simulink model "Rebuild"  (R2024b)
settings: Solver=VariableStepAuto  StartTime=0.0  StopTime=12  RelTol=1e-3
values from neighbouring files (symbols this model uses):
  A = 1.1    [RT14e_Parameters.m]    (also in RT15e_Parameters.m = 1.088; RT15evo_Parameters.m = 1.088)
  Aero_balance = 55    [RT14e_Parameters.m]    (also in RT15e_Parameters.m; RT15evo_Parameters.m)
  Aeromaps_ON = 0    [SIM_setup.m]
  air_density = 1.2    [SIM_setup.m]
  Balance_FW = Data_FW_STD(1:end,2)    [RT15e_Parameters.m]    (also in RT15evo_Parameters.m)
  Balance_R_11 = Data_R_11(1:end,2)    [RT15e_Parameters.m]    (also in RT15evo_Parameters.m)
  Br_coef_of_friction_F = 0.33    [RT14e_Parameters.m]    (also in RT15e_Parameters.m; RT15evo_Parameters.m)
  Br_coef_of_friction_R = 0.33    [RT14e_Parameters.m]    (also in RT15e_Parameters.m; RT15evo_Parameters.m)
  Br_pistons_area_F = 3617.26/1e6    (= 0.00361726)    [RT14e_Parameters.m]    (also in RT15e_Parameters.m; RT15evo_Parameters.m)
  Br_pistons_area_R = 2026.83/1e6    (= 0.00202683)    [RT14e_Parameters.m]    (also in RT15e_Parameters.m; RT15evo_Parameters.m)
  CdA = 1.31*A    (= 1.441)    [RT14e_Parameters.m]    (also in RT15e_Parameters.m = 1.700544; RT15evo_Parameters.m = 1.700544)
  CdA_FW = Data_FW_STD(1:end,3)    [RT15e_Parameters.m]    (also in RT15evo_Parameters.m)
  CdA_R_11 = Data_R_11(1:end,3)    [RT15e_Parameters.m]    (also in RT15evo_Parameters.m)
  ClA = 3.3*A    (= 3.63)    [RT14e_Parameters.m]    (also in RT15e_Parameters.m = 4.36288; RT15evo_Parameters.m = 4.36288)
  ClA_FW = Data_FW_STD(1:end,4)    [RT15e_Parameters.m]    (also in RT15evo_Parameters.m)
  ClA_R_11 = Data_R_11(1:end,4)    [RT15e_Parameters.m]    (also in RT15evo_Parameters.m)
  CoG_z = 0.35    [RT14e_Parameters.m]    (also in RT15e_Parameters.m = 0.28495; RT15evo_Parameters.m = 0.28495)
  Default_Fz_FL = Default_Fz_F/2 + (Default_Fz_F*CoG_y/Track_Front)    [RT14e_Parameters.m]    (also in RT15e_Parameters.m; RT15evo_Parameters.m)
  Default_Fz_FR = Default_Fz_F/2 - (Default_Fz_F*CoG_y/Track_Front)    [RT14e_Parameters.m]    (also in RT15e_Parameters.m; RT15evo_Parameters.m)
  Default_Fz_RL = Default_Fz_R/2 + (Default_Fz_R*CoG_y/Track_Rear)    [RT14e_Parameters.m]    (also in RT15e_Parameters.m; RT15evo_Parameters.m)
  Default_Fz_RR = Default_Fz_R/2 - (Default_Fz_R*CoG_y/Track_Rear)    [RT14e_Parameters.m]    (also in RT15e_Parameters.m; RT15evo_Parameters.m)
  Effective_br_disk_r_F = 0.0905    [RT14e_Parameters.m]    (also in RT15e_Parameters.m; RT15evo_Parameters.m)
  Effective_br_disk_r_R = 0.0895    [RT14e_Parameters.m]    (also in RT15e_Parameters.m; RT15evo_Parameters.m)
  Front_brake_balance = 0.0    (= 0)    [RT14e_Parameters.m]    (also in RT15e_Parameters.m; RT15evo_Parameters.m)
  Front_brake_pump_area = 153.94    [RT14e_Parameters.m]    (also in RT15e_Parameters.m; RT15evo_Parameters.m)
  Front_desired_brake_p_balance = 0.6    [RT14e_Parameters.m]    (also in RT15e_Parameters.m; RT15evo_Parameters.m)
  FW_Setup = Data_FW_STD(1:end,1)    [RT15e_Parameters.m]    (also in RT15evo_Parameters.m)
  Fx = Data_Fx(2:end,3:end)    [RT14e_Parameters.m]    (also in RT15e_Parameters.m; RT15evo_Parameters.m)
  Fy = Data_Fy(2:end,3:end)    [RT14e_Parameters.m]    (also in RT15e_Parameters.m; RT15evo_Parameters.m)
  Fz = Data_Fy(2:end,2)    [RT14e_Parameters.m]    (also in RT15e_Parameters.m; RT15evo_Parameters.m)
  g = 9.81    [SIM_setup.m]
  Gear_ratio = 12.9    [RT14e_Parameters.m]    (also in RT15e_Parameters.m; RT15evo_Parameters.m)
  Iz_wehicle = 120    [RT14e_Parameters.m]    (also in RT15e_Parameters.m; RT15evo_Parameters.m)
  Iz_wheel = 0.15    [RT14e_Parameters.m]    (also in RT15e_Parameters.m; RT15evo_Parameters.m)
  Lf = Wheelbase - CoG_x    (= 0.77)    [RT14e_Parameters.m]    (also in RT15e_Parameters.m = 0.7504; RT15evo_Parameters.m = 0.7504)
  LLTD = 0.45    [RT14e_Parameters.m]    (also in RT15e_Parameters.m = 0.55; RT15evo_Parameters.m = 0.55)
  Lock_brake_balance = false    [RT14e_Parameters.m]    (also in RT15e_Parameters.m; RT15evo_Parameters.m)
  Lr = Wheelbase - Lf    (= 0.755)    [RT14e_Parameters.m]    (also in RT15e_Parameters.m = 0.7746; RT15evo_Parameters.m = 0.7746)
  Mass = Vehicle_mass + Driver_mass    (= 290)    [RT14e_Parameters.m]    (also in RT15e_Parameters.m = 265; RT15evo_Parameters.m)
  Motor_maximum_power = 35366    [RT14e_Parameters.m]    (also in RT15e_Parameters.m; RT15evo_Parameters.m)
  RB_torque_setting_1 = -2    [RT14e_Parameters.m]    (also in RT15e_Parameters.m; RT15evo_Parameters.m)
  RB_torque_setting_10 = -20    [RT14e_Parameters.m]    (also in RT15e_Parameters.m; RT15evo_Parameters.m)
  RB_torque_setting_2 = -4    [RT14e_Parameters.m]    (also in RT15e_Parameters.m; RT15evo_Parameters.m)
  RB_torque_setting_3 = -6    [RT14e_Parameters.m]    (also in RT15e_Parameters.m; RT15evo_Parameters.m)
  RB_torque_setting_4 = -8    [RT14e_Parameters.m]    (also in RT15e_Parameters.m; RT15evo_Parameters.m)
  RB_torque_setting_5 = -10    [RT14e_Parameters.m]    (also in RT15e_Parameters.m; RT15evo_Parameters.m)
  RB_torque_setting_6 = -12    [RT14e_Parameters.m]    (also in RT15e_Parameters.m; RT15evo_Parameters.m)
  RB_torque_setting_7 = -14    [RT14e_Parameters.m]    (also in RT15e_Parameters.m; RT15evo_Parameters.m)
  RB_torque_setting_8 = -16    [RT14e_Parameters.m]    (also in RT15e_Parameters.m; RT15evo_Parameters.m)
  RB_torque_setting_9 = -18    [RT14e_Parameters.m]    (also in RT15e_Parameters.m; RT15evo_Parameters.m)
  Rear_brake_pump_area = 198.56    [RT14e_Parameters.m]    (also in RT15e_Parameters.m; RT15evo_Parameters.m)
  Roll_Angle_11 = Data_R_11(1:end,1)    [RT15e_Parameters.m]    (also in RT15evo_Parameters.m)
  SA = Data_Fy(1,3:end)    [RT14e_Parameters.m]    (also in RT15e_Parameters.m; RT15evo_Parameters.m)
  SR = Data_Fx(1,3:end)    [RT14e_Parameters.m]    (also in RT15e_Parameters.m; RT15evo_Parameters.m)
  start_acc_x = double(start_acc_x_ts.Data)    [SIM_setup.m]
  start_acc_y = double(start_acc_y_ts.Data)    [SIM_setup.m]
  start_time = 1188    [SIM_setup.m]
  start_velocity_x = double(start_velocity_x_ts.Data)    [SIM_setup.m]
  start_velocity_y = double(start_velocity_y_ts.Data)    [SIM_setup.m]
  start_yaw_acc = double(start_yaw_acc_ts.Data)    [SIM_setup.m]
  start_yaw_rate = double(start_yaw_rate_ts.Data)    [SIM_setup.m]
  Static_Camber_FL = 0    [RT14e_Parameters.m]    (also in RT15e_Parameters.m; RT15evo_Parameters.m)
  Static_Camber_FR = 0    [RT14e_Parameters.m]    (also in RT15e_Parameters.m; RT15evo_Parameters.m)
  Static_Camber_RL = 0    [RT14e_Parameters.m]    (also in RT15e_Parameters.m; RT15evo_Parameters.m)
  Static_Camber_RR = 0    [RT14e_Parameters.m]    (also in RT15e_Parameters.m; RT15evo_Parameters.m)
  Static_Toe_FL = 0    [RT14e_Parameters.m]    (also in RT15e_Parameters.m; RT15evo_Parameters.m)
  Static_Toe_FR = 0    [RT14e_Parameters.m]    (also in RT15e_Parameters.m; RT15evo_Parameters.m)
  Static_Toe_RL = 0    [RT14e_Parameters.m]    (also in RT15e_Parameters.m; RT15evo_Parameters.m)
  Static_Toe_RR = 0    [RT14e_Parameters.m]    (also in RT15e_Parameters.m; RT15evo_Parameters.m)
  Steering_Angle_FL = Data_Steering(1:end,2)    [RT14e_Parameters.m]    (also in RT15e_Parameters.m; RT15evo_Parameters.m)
  Steering_Angle_FR = Data_Steering(1:end,3)    [RT14e_Parameters.m]    (also in RT15e_Parameters.m; RT15evo_Parameters.m)
  Steering_Wheel_Angle = Data_Steering(1:end,1)    [RT14e_Parameters.m]    (also in RT15e_Parameters.m; RT15evo_Parameters.m)
  Tire_radius = 0.203    [RT14e_Parameters.m]    (also in RT15e_Parameters.m; RT15evo_Parameters.m)
  Torque_limit_2 = Motor_maximum_torque*0.2    (= 5.82)    [RT14e_Parameters.m]    (also in RT15e_Parameters.m; RT15evo_Parameters.m)
  Torque_limit_3 = Motor_maximum_torque*0.3    (= 8.73)    [RT14e_Parameters.m]    (also in RT15e_Parameters.m; RT15evo_Parameters.m)
  Torque_limit_4 = Motor_maximum_torque*0.4    (= 11.64)    [RT14e_Parameters.m]    (also in RT15e_Parameters.m; RT15evo_Parameters.m)
  Torque_limit_5 = Motor_maximum_torque*0.5    (= 14.55)    [RT14e_Parameters.m]    (also in RT15e_Parameters.m; RT15evo_Parameters.m)
  Torque_limit_6 = Motor_maximum_torque*0.6    (= 17.46)    [RT14e_Parameters.m]    (also in RT15e_Parameters.m; RT15evo_Parameters.m)
  Torque_limit_7 = Motor_maximum_torque*0.7    (= 20.37)    [RT14e_Parameters.m]    (also in RT15e_Parameters.m; RT15evo_Parameters.m)
  Torque_limit_8 = Motor_maximum_torque*0.8    (= 23.28)    [RT14e_Parameters.m]    (also in RT15e_Parameters.m; RT15evo_Parameters.m)
  Torque_limit_9 = 29.1    [RT14e_Parameters.m]    (also in RT15e_Parameters.m; RT15evo_Parameters.m)
  Torque_limit_max = Motor_maximum_torque    (= 29.1)    [RT14e_Parameters.m]    (also in RT15e_Parameters.m; RT15evo_Parameters.m)
  Torque_limit_min = Motor_maximum_torque*0.1    (= 2.91)    [RT14e_Parameters.m]    (also in RT15e_Parameters.m; RT15evo_Parameters.m)
  Torque_limit_set = 10    [RT14e_Parameters.m]    (also in RT15e_Parameters.m; RT15evo_Parameters.m)
  Track_Front = 1.2    [RT14e_Parameters.m]    (also in RT15e_Parameters.m; RT15evo_Parameters.m)
  Track_Rear = 1.18    [RT14e_Parameters.m]    (also in RT15e_Parameters.m; RT15evo_Parameters.m)
  TV_ON = 0    [SIM_setup.m]
  TV_RB_understeer_gradient_1 = -0.5    [RT14e_Parameters.m]    (also in RT15e_Parameters.m; RT15evo_Parameters.m)
  TV_RB_understeer_gradient_10 = 0.005    [RT14e_Parameters.m]    (also in RT15e_Parameters.m; RT15evo_Parameters.m)
  TV_RB_understeer_gradient_2 = -0.1    [RT14e_Parameters.m]    (also in RT15e_Parameters.m; RT15evo_Parameters.m)
  TV_RB_understeer_gradient_3 = 0.08    [RT14e_Parameters.m]    (also in RT15e_Parameters.m; RT15evo_Parameters.m)
  TV_RB_understeer_gradient_4 = 0.06    [RT14e_Parameters.m]    (also in RT15e_Parameters.m; RT15evo_Parameters.m)
  TV_RB_understeer_gradient_5 = 0.05    [RT14e_Parameters.m]    (also in RT15e_Parameters.m; RT15evo_Parameters.m)
  TV_RB_understeer_gradient_6 = 0.04    [RT14e_Parameters.m]    (also in RT15e_Parameters.m; RT15evo_Parameters.m)
  TV_RB_understeer_gradient_7 = 0.03    [RT14e_Parameters.m]    (also in RT15e_Parameters.m; RT15evo_Parameters.m)
  TV_RB_understeer_gradient_8 = 0.02    [RT14e_Parameters.m]    (also in RT15e_Parameters.m; RT15evo_Parameters.m)
  TV_RB_understeer_gradient_9 = 0.01    [RT14e_Parameters.m]    (also in RT15e_Parameters.m; RT15evo_Parameters.m)
  TV_understeer_gradient_1 = -0.5    [RT14e_Parameters.m]    (also in RT15e_Parameters.m; RT15evo_Parameters.m)
  TV_understeer_gradient_10 = 0.002    [RT14e_Parameters.m]    (also in RT15e_Parameters.m; RT15evo_Parameters.m)
  TV_understeer_gradient_2 = -0.1    [RT14e_Parameters.m]    (also in RT15e_Parameters.m; RT15evo_Parameters.m)
  TV_understeer_gradient_3 = 0.06    [RT14e_Parameters.m]    (also in RT15e_Parameters.m; RT15evo_Parameters.m)
  TV_understeer_gradient_4 = 0.05    [RT14e_Parameters.m]    (also in RT15e_Parameters.m; RT15evo_Parameters.m)
  TV_understeer_gradient_5 = 0.04    [RT14e_Parameters.m]    (also in RT15e_Parameters.m; RT15evo_Parameters.m)
  TV_understeer_gradient_6 = 0.03    [RT14e_Parameters.m]    (also in RT15e_Parameters.m; RT15evo_Parameters.m)
  TV_understeer_gradient_7 = 0.02    [RT14e_Parameters.m]    (also in RT15e_Parameters.m; RT15evo_Parameters.m)
  TV_understeer_gradient_8 = 0.01    [RT14e_Parameters.m]    (also in RT15e_Parameters.m; RT15evo_Parameters.m)
  TV_understeer_gradient_9 = 0.005    [RT14e_Parameters.m]    (also in RT15e_Parameters.m; RT15evo_Parameters.m)
  Vx_APPS_ON = 1    [SIM_setup.m]
  Wheel_rolling_resistance = 0.055    [RT14e_Parameters.m]    (also in RT15e_Parameters.m; RT15evo_Parameters.m)
  Wheelbase = 1.525    [RT14e_Parameters.m]    (also in RT15e_Parameters.m; RT15evo_Parameters.m)
undefined symbols (not defined in the file or in its folder): Actual_Torque_Value_RL, Actual_Torque_Value_RR, aero_balance, APPS, Brake_Pressure_Front, Brake_Pressure_Rear, Cl, lateral_load_transfer_distribution, maths_GPS_Velocity, Max_Torque, rad, s, Steering_position, tire_radius, wheel_base, Wheel_Speed_RL, Wheel_Speed_RR, Xsens_MTI_670_accX, Xsens_MTI_670_accY, Xsens_MTI_670_gyrZ
libraries: simulink x30, simulink_extras x11, slpidlib x9, dspstat3 x4, slrealtimeloglib x1, aerolibconvert2 x1
(part 4 of 6)

== system Rebuild/Main/Powertrain/Motors/Control Algorithms/ABS/ABS_RR ==
  Torque IN : Inport
  Slip_Ratio : Inport  Port=2
  Constant : Constant  Value=0.1
  Constant1 : Constant  Value=0.1
  Constant2 : Constant  Value=0.2
  Constant3 : Constant  Value=0
  Constant4 : Constant
  Gain : Gain  Gain=-1
  PID Controller : slpidlib/PID Controller  Controller=PI  Form=Ideal  TimeDomain=Continuous-time  UseExternalTs=off  SampleTime=-1  IntegratorMethod=Forward Euler  FilterMethod=Forward Euler  ControllerParametersSource=internal  P=100  I=10  UseKiTs=on  D=1  UseExternalDerivativeSource=off  N=100  UseFilter=on  TunerSelectOption=Transfer Function Based (PID Tuner App)  InitialConditionSource=internal  InitialConditionForIntegrator=0  InitialConditionForFilter=0  DifferentiatorICPrevScaledInput=0  ExternalReset=none  TrackingMode=off  Kt=1  LimitOutput=off  SatLimitsSource=internal  UpperSaturationLimit=inf  LowerSaturationLimit=-inf  LinearizeAsGain=on  AntiWindupMode=none  Kb=1  LimitIntegrator=off  UpperIntegratorSaturationLimit=inf  LowerIntegratorSaturationLimit=-inf  POutMin=[]  POutMax=[]  IOutMin=[]  IOutMax=[]  DOutMin=[]  DOutMax=[]  NOutMin=[]  NOutMax=[]  SumOutMin=[]  SumOutMax=[]  SaturationOutMin=[]  SaturationOutMax=[]  PParamMin=[]  PParamMax=[]  IParamMin=[]  IParamMax=[]  DParamMin=[]  DParamMax=[]  NParamMin=[]  NParamMax=[]  KbParamMin=[]  KbParamMax=[]  KtParamMin=[]  KtParamMax=[]  KbOutMin=[]  KbOutMax=[]  KtOutMin=[]  KtOutMax=[]  IntegratorOutMin=[]  IntegratorOutMax=[]  FilterOutMin=[]  FilterOutMax=[]  SumI1OutMin=[]  SumI1OutMax=[]  SumI2OutMin=[]  SumI2OutMax=[]  SumI3OutMin=[]  SumI3OutMax=[]  SumI4OutMin=[]  SumI4OutMax=[]  SumDOutMin=[]  SumDOutMax=[]  DifferentiatorOutMin=[]  DifferentiatorOutMax=[]  FilterDiffOutCoefMin=[]  FilterDiffOutCoefMax=[]  ReciprocalOutMin=[]  ReciprocalOutMax=[]  SumDenOutMin=[]  SumDenOutMax=[]  SumNumOutMin=[]  SumNumOutMax=[]  DivideOutMin=[]  DivideOutMax=[]  UdiffTsProdOutMin=[]  UdiffTsProdOutMax=[]  NTsProdOutMin=[]  NTsProdOutMax=[]  UintegralTsProdOutMin=[]  UintegralTsProdOutMax=[]  UngainTsProdOutMin=[]  UngainTsProdOutMax=[]  ClampingZeroOutDataTypeStr=Inherit: Inherit via back propagation  ClampingZeroOutMin=[]  ClampingZeroOutMax=[]  FilterDenConstantOutDataTypeStr=Inherit: Inherit via back propagation  FilterDenConstantOutMin=[]  FilterDenConstantOutMax=[]  PCopyOutDataTypeStr=Inherit: Inherit via back propagation  PCopyOutMin=[]  PCopyOutMax=[]  NCopyOutDataTypeStr=Inherit: Inherit via back propagation  NCopyOutMin=[]  NCopyOutMax=[]  IntegratorContinuousStateAttributes=''  IntegratorStateMustResolveToSignalObject=off  IntegratorRTWStateStorageClass=Auto  FilterContinuousStateAttributes=''  FilterStateMustResolveToSignalObject=off  FilterRTWStateStorageClass=Auto  ParallelPVariant=Passthrough  IdealPVariant=InternalParameters  IVariant=InternalParameters  DVariant=Disabled  IntegratorVariant=Continuous  SatVariant=Disabled  AWVariant=Passthrough  PCopyVariant=Disabled  TRVariant=Disabled  FdbkBlocksVariant=Forward  IdealPFdbkVariant=Disabled  SatFdbkVariant=Disabled  DerivativeFilterVariant=Disabled  NVariant=Disabled  NCopyVariant=Disabled_SignalSpec  FilterICVariant=Disabled  IntegratorICVariant=InternalICs  ExternalResetVariant=Disabled  TRSumVariant=Passthrough  SumFdbkVariant=Disabled  SumVariant=Sum_PI  TsampFilterVariant=InternalTs  TsampNgainVariant=Passthrough  TsampIntegralVariant=Disabled_SignalSpec  ExternalSaturationOutDataTypeStr=Inherit: Same as second input  DerivativeSourceVariant=Disabled  PreIntVariant=InternalPreInt
  Product : Product
  Relational Operator : RelationalOperator  Operator=<=  OutDataTypeStr=boolean  RndMeth=Simplest  InputSameDT=off
  Sum1 : Sum  Inputs=|++
  Switch : Switch  Criteria=u2 > Threshold  SaturateOnIntegerOverflow=off  InputSameDT=off
  Switch1 : Switch  Criteria=u2 > Threshold  SaturateOnIntegerOverflow=off  InputSameDT=off
  Switch2 : Switch  Criteria=u2 > Threshold  SaturateOnIntegerOverflow=off  InputSameDT=off
  ABS Torque OUT : Outport
  wires:
  Product/1 -> ABS Torque OUT/1  "Torq OUT"
  Switch/1 -> Sum1/2  "Ref Slip Ratio"
  Constant/1 -> Relational Operator/1
  Sum1/1 -> Switch1/1  "Slip Ratio Delta"
  Switch1/1 -> PID Controller/1
  PID Controller/1 -> Switch2/1
  Constant2/1 -> Switch/3
  Gain/1 -> Relational Operator/2
  Switch2/1 -> Product/2
  Constant4/1 -> Switch2/3
  Torque IN/1 -> Product/1  "Torque IN"
  Constant1/1 -> Switch/2, Switch/1
  Constant3/1 -> Switch1/3
  Relational Operator/1 -> Switch2/2, Switch1/2
  Slip_Ratio/1 -> Gain/1, Sum1/1  "Slip Ratio"

== system Rebuild/Main/Powertrain/Motors/Control Algorithms/ABS1/ABS_FL1 ==
  Torque IN : Inport
  Slip_Ratio : Inport  Port=2
  Constant1 : Constant  Value=0.15
  Constant2 : Constant  Value=0.3
  Gain : Gain  Gain=-1
  PID Controller : slpidlib/PID Controller  Controller=PI  Form=Ideal  TimeDomain=Continuous-time  UseExternalTs=off  SampleTime=-1  IntegratorMethod=Forward Euler  FilterMethod=Forward Euler  ControllerParametersSource=internal  P=50  I=2.5  UseKiTs=on  D=1  UseExternalDerivativeSource=off  N=100  UseFilter=on  TunerSelectOption=Transfer Function Based (PID Tuner App)  InitialConditionSource=internal  InitialConditionForIntegrator=0  InitialConditionForFilter=0  DifferentiatorICPrevScaledInput=0  ExternalReset=none  TrackingMode=off  Kt=1  LimitOutput=off  SatLimitsSource=internal  UpperSaturationLimit=inf  LowerSaturationLimit=-inf  LinearizeAsGain=on  AntiWindupMode=none  Kb=1  LimitIntegrator=off  UpperIntegratorSaturationLimit=inf  LowerIntegratorSaturationLimit=-inf  POutMin=[]  POutMax=[]  IOutMin=[]  IOutMax=[]  DOutMin=[]  DOutMax=[]  NOutMin=[]  NOutMax=[]  SumOutMin=[]  SumOutMax=[]  SaturationOutMin=[]  SaturationOutMax=[]  PParamMin=[]  PParamMax=[]  IParamMin=[]  IParamMax=[]  DParamMin=[]  DParamMax=[]  NParamMin=[]  NParamMax=[]  KbParamMin=[]  KbParamMax=[]  KtParamMin=[]  KtParamMax=[]  KbOutMin=[]  KbOutMax=[]  KtOutMin=[]  KtOutMax=[]  IntegratorOutMin=[]  IntegratorOutMax=[]  FilterOutMin=[]  FilterOutMax=[]  SumI1OutMin=[]  SumI1OutMax=[]  SumI2OutMin=[]  SumI2OutMax=[]  SumI3OutMin=[]  SumI3OutMax=[]  SumI4OutMin=[]  SumI4OutMax=[]  SumDOutMin=[]  SumDOutMax=[]  DifferentiatorOutMin=[]  DifferentiatorOutMax=[]  FilterDiffOutCoefMin=[]  FilterDiffOutCoefMax=[]  ReciprocalOutMin=[]  ReciprocalOutMax=[]  SumDenOutMin=[]  SumDenOutMax=[]  SumNumOutMin=[]  SumNumOutMax=[]  DivideOutMin=[]  DivideOutMax=[]  UdiffTsProdOutMin=[]  UdiffTsProdOutMax=[]  NTsProdOutMin=[]  NTsProdOutMax=[]  UintegralTsProdOutMin=[]  UintegralTsProdOutMax=[]  UngainTsProdOutMin=[]  UngainTsProdOutMax=[]  ClampingZeroOutDataTypeStr=Inherit: Inherit via back propagation  ClampingZeroOutMin=[]  ClampingZeroOutMax=[]  FilterDenConstantOutDataTypeStr=Inherit: Inherit via back propagation  FilterDenConstantOutMin=[]  FilterDenConstantOutMax=[]  PCopyOutDataTypeStr=Inherit: Inherit via back propagation  PCopyOutMin=[]  PCopyOutMax=[]  NCopyOutDataTypeStr=Inherit: Inherit via back propagation  NCopyOutMin=[]  NCopyOutMax=[]  IntegratorContinuousStateAttributes=''  IntegratorStateMustResolveToSignalObject=off  IntegratorRTWStateStorageClass=Auto  FilterContinuousStateAttributes=''  FilterStateMustResolveToSignalObject=off  FilterRTWStateStorageClass=Auto  ParallelPVariant=Passthrough  IdealPVariant=InternalParameters  IVariant=InternalParameters  DVariant=Disabled  IntegratorVariant=Continuous  SatVariant=Disabled  AWVariant=Passthrough  PCopyVariant=Disabled  TRVariant=Disabled  FdbkBlocksVariant=Forward  IdealPFdbkVariant=Disabled  SatFdbkVariant=Disabled  DerivativeFilterVariant=Disabled  NVariant=Disabled  NCopyVariant=Disabled_SignalSpec  FilterICVariant=Disabled  IntegratorICVariant=InternalICs  ExternalResetVariant=Disabled  TRSumVariant=Passthrough  SumFdbkVariant=Disabled  SumVariant=Sum_PI  TsampFilterVariant=InternalTs  TsampNgainVariant=Passthrough  TsampIntegralVariant=Disabled_SignalSpec  ExternalSaturationOutDataTypeStr=Inherit: Same as second input  DerivativeSourceVariant=Disabled  PreIntVariant=InternalPreInt
  Product : Product
  Saturation : Saturate  UpperLimit=5  LowerLimit=-5
  Scope : Scope
  Sum1 : Sum  Inputs=|++
  Switch : Switch  Criteria=u2 > Threshold  SaturateOnIntegerOverflow=off  InputSameDT=off
  ABS Torque OUT : Outport
  wires:
  Switch/1 -> Sum1/2  "Ref Slip Ratio"
  Product/1 -> ABS Torque OUT/1  "Torq OUT"
  PID Controller/1 -> Scope/1, Saturation/1
  Slip_Ratio/1 -> Gain/1  "Slip Ratio"
  Constant1/1 -> Switch/2, Switch/1
  Torque IN/1 -> Product/1  "Torque IN"
  Sum1/1 -> PID Controller/1  "Slip Ratio Delta"
  Constant2/1 -> Switch/3
  Saturation/1 -> Product/2
  Gain/1 -> Sum1/1

== system Rebuild/Main/Powertrain/Motors/Control Algorithms/ABS1/ABS_FR1 ==
  Torque IN : Inport
  Slip_Ratio : Inport  Port=2
  Constant1 : Constant  Value=0.15
  Constant2 : Constant  Value=0.3
  Gain : Gain  Gain=-1
  PID Controller : slpidlib/PID Controller  Controller=PI  Form=Ideal  TimeDomain=Continuous-time  UseExternalTs=off  SampleTime=-1  IntegratorMethod=Forward Euler  FilterMethod=Forward Euler  ControllerParametersSource=internal  P=50  I=2.5  UseKiTs=on  D=1  UseExternalDerivativeSource=off  N=100  UseFilter=on  TunerSelectOption=Transfer Function Based (PID Tuner App)  InitialConditionSource=internal  InitialConditionForIntegrator=0  InitialConditionForFilter=0  DifferentiatorICPrevScaledInput=0  ExternalReset=none  TrackingMode=off  Kt=1  LimitOutput=off  SatLimitsSource=internal  UpperSaturationLimit=inf  LowerSaturationLimit=-inf  LinearizeAsGain=on  AntiWindupMode=none  Kb=1  LimitIntegrator=off  UpperIntegratorSaturationLimit=inf  LowerIntegratorSaturationLimit=-inf  POutMin=[]  POutMax=[]  IOutMin=[]  IOutMax=[]  DOutMin=[]  DOutMax=[]  NOutMin=[]  NOutMax=[]  SumOutMin=[]  SumOutMax=[]  SaturationOutMin=[]  SaturationOutMax=[]  PParamMin=[]  PParamMax=[]  IParamMin=[]  IParamMax=[]  DParamMin=[]  DParamMax=[]  NParamMin=[]  NParamMax=[]  KbParamMin=[]  KbParamMax=[]  KtParamMin=[]  KtParamMax=[]  KbOutMin=[]  KbOutMax=[]  KtOutMin=[]  KtOutMax=[]  IntegratorOutMin=[]  IntegratorOutMax=[]  FilterOutMin=[]  FilterOutMax=[]  SumI1OutMin=[]  SumI1OutMax=[]  SumI2OutMin=[]  SumI2OutMax=[]  SumI3OutMin=[]  SumI3OutMax=[]  SumI4OutMin=[]  SumI4OutMax=[]  SumDOutMin=[]  SumDOutMax=[]  DifferentiatorOutMin=[]  DifferentiatorOutMax=[]  FilterDiffOutCoefMin=[]  FilterDiffOutCoefMax=[]  ReciprocalOutMin=[]  ReciprocalOutMax=[]  SumDenOutMin=[]  SumDenOutMax=[]  SumNumOutMin=[]  SumNumOutMax=[]  DivideOutMin=[]  DivideOutMax=[]  UdiffTsProdOutMin=[]  UdiffTsProdOutMax=[]  NTsProdOutMin=[]  NTsProdOutMax=[]  UintegralTsProdOutMin=[]  UintegralTsProdOutMax=[]  UngainTsProdOutMin=[]  UngainTsProdOutMax=[]  ClampingZeroOutDataTypeStr=Inherit: Inherit via back propagation  ClampingZeroOutMin=[]  ClampingZeroOutMax=[]  FilterDenConstantOutDataTypeStr=Inherit: Inherit via back propagation  FilterDenConstantOutMin=[]  FilterDenConstantOutMax=[]  PCopyOutDataTypeStr=Inherit: Inherit via back propagation  PCopyOutMin=[]  PCopyOutMax=[]  NCopyOutDataTypeStr=Inherit: Inherit via back propagation  NCopyOutMin=[]  NCopyOutMax=[]  IntegratorContinuousStateAttributes=''  IntegratorStateMustResolveToSignalObject=off  IntegratorRTWStateStorageClass=Auto  FilterContinuousStateAttributes=''  FilterStateMustResolveToSignalObject=off  FilterRTWStateStorageClass=Auto  ParallelPVariant=Passthrough  IdealPVariant=InternalParameters  IVariant=InternalParameters  DVariant=Disabled  IntegratorVariant=Continuous  SatVariant=Disabled  AWVariant=Passthrough  PCopyVariant=Disabled  TRVariant=Disabled  FdbkBlocksVariant=Forward  IdealPFdbkVariant=Disabled  SatFdbkVariant=Disabled  DerivativeFilterVariant=Disabled  NVariant=Disabled  NCopyVariant=Disabled_SignalSpec  FilterICVariant=Disabled  IntegratorICVariant=InternalICs  ExternalResetVariant=Disabled  TRSumVariant=Passthrough  SumFdbkVariant=Disabled  SumVariant=Sum_PI  TsampFilterVariant=InternalTs  TsampNgainVariant=Passthrough  TsampIntegralVariant=Disabled_SignalSpec  ExternalSaturationOutDataTypeStr=Inherit: Same as second input  DerivativeSourceVariant=Disabled  PreIntVariant=InternalPreInt
  Product : Product
  Saturation : Saturate  UpperLimit=5  LowerLimit=-5
  Scope : Scope
  Sum1 : Sum  Inputs=|++
  Switch : Switch  Criteria=u2 > Threshold  SaturateOnIntegerOverflow=off  InputSameDT=off
  ABS Torque OUT : Outport
  wires:
  Constant1/1 -> Switch/2, Switch/1
  Switch/1 -> Sum1/2  "Ref Slip Ratio"
  Constant2/1 -> Switch/3
  Sum1/1 -> PID Controller/1  "Slip Ratio Delta"
  Torque IN/1 -> Product/1  "Torque IN"
  Product/1 -> ABS Torque OUT/1  "Torq OUT"
  Slip_Ratio/1 -> Gain/1  "Slip Ratio"
  PID Controller/1 -> Scope/1, Saturation/1
  Saturation/1 -> Product/2
  Gain/1 -> Sum1/1

== system Rebuild/Main/Powertrain/Motors/Control Algorithms/ABS1/ABS_RL1 ==
  Torque IN : Inport
  Slip_Ratio : Inport  Port=2
  Constant1 : Constant  Value=0.15
  Constant2 : Constant  Value=0.3
  Gain : Gain  Gain=-1
  PID Controller : slpidlib/PID Controller  Controller=PI  Form=Ideal  TimeDomain=Continuous-time  UseExternalTs=off  SampleTime=-1  IntegratorMethod=Forward Euler  FilterMethod=Forward Euler  ControllerParametersSource=internal  P=50  I=2.5  UseKiTs=on  D=1  UseExternalDerivativeSource=off  N=100  UseFilter=on  TunerSelectOption=Transfer Function Based (PID Tuner App)  InitialConditionSource=internal  InitialConditionForIntegrator=0  InitialConditionForFilter=0  DifferentiatorICPrevScaledInput=0  ExternalReset=none  TrackingMode=off  Kt=1  LimitOutput=off  SatLimitsSource=internal  UpperSaturationLimit=inf  LowerSaturationLimit=-inf  LinearizeAsGain=on  AntiWindupMode=none  Kb=1  LimitIntegrator=off  UpperIntegratorSaturationLimit=inf  LowerIntegratorSaturationLimit=-inf  POutMin=[]  POutMax=[]  IOutMin=[]  IOutMax=[]  DOutMin=[]  DOutMax=[]  NOutMin=[]  NOutMax=[]  SumOutMin=[]  SumOutMax=[]  SaturationOutMin=[]  SaturationOutMax=[]  PParamMin=[]  PParamMax=[]  IParamMin=[]  IParamMax=[]  DParamMin=[]  DParamMax=[]  NParamMin=[]  NParamMax=[]  KbParamMin=[]  KbParamMax=[]  KtParamMin=[]  KtParamMax=[]  KbOutMin=[]  KbOutMax=[]  KtOutMin=[]  KtOutMax=[]  IntegratorOutMin=[]  IntegratorOutMax=[]  FilterOutMin=[]  FilterOutMax=[]  SumI1OutMin=[]  SumI1OutMax=[]  SumI2OutMin=[]  SumI2OutMax=[]  SumI3OutMin=[]  SumI3OutMax=[]  SumI4OutMin=[]  SumI4OutMax=[]  SumDOutMin=[]  SumDOutMax=[]  DifferentiatorOutMin=[]  DifferentiatorOutMax=[]  FilterDiffOutCoefMin=[]  FilterDiffOutCoefMax=[]  ReciprocalOutMin=[]  ReciprocalOutMax=[]  SumDenOutMin=[]  SumDenOutMax=[]  SumNumOutMin=[]  SumNumOutMax=[]  DivideOutMin=[]  DivideOutMax=[]  UdiffTsProdOutMin=[]  UdiffTsProdOutMax=[]  NTsProdOutMin=[]  NTsProdOutMax=[]  UintegralTsProdOutMin=[]  UintegralTsProdOutMax=[]  UngainTsProdOutMin=[]  UngainTsProdOutMax=[]  ClampingZeroOutDataTypeStr=Inherit: Inherit via back propagation  ClampingZeroOutMin=[]  ClampingZeroOutMax=[]  FilterDenConstantOutDataTypeStr=Inherit: Inherit via back propagation  FilterDenConstantOutMin=[]  FilterDenConstantOutMax=[]  PCopyOutDataTypeStr=Inherit: Inherit via back propagation  PCopyOutMin=[]  PCopyOutMax=[]  NCopyOutDataTypeStr=Inherit: Inherit via back propagation  NCopyOutMin=[]  NCopyOutMax=[]  IntegratorContinuousStateAttributes=''  IntegratorStateMustResolveToSignalObject=off  IntegratorRTWStateStorageClass=Auto  FilterContinuousStateAttributes=''  FilterStateMustResolveToSignalObject=off  FilterRTWStateStorageClass=Auto  ParallelPVariant=Passthrough  IdealPVariant=InternalParameters  IVariant=InternalParameters  DVariant=Disabled  IntegratorVariant=Continuous  SatVariant=Disabled  AWVariant=Passthrough  PCopyVariant=Disabled  TRVariant=Disabled  FdbkBlocksVariant=Forward  IdealPFdbkVariant=Disabled  SatFdbkVariant=Disabled  DerivativeFilterVariant=Disabled  NVariant=Disabled  NCopyVariant=Disabled_SignalSpec  FilterICVariant=Disabled  IntegratorICVariant=InternalICs  ExternalResetVariant=Disabled  TRSumVariant=Passthrough  SumFdbkVariant=Disabled  SumVariant=Sum_PI  TsampFilterVariant=InternalTs  TsampNgainVariant=Passthrough  TsampIntegralVariant=Disabled_SignalSpec  ExternalSaturationOutDataTypeStr=Inherit: Same as second input  DerivativeSourceVariant=Disabled  PreIntVariant=InternalPreInt
  Product : Product
  Saturation : Saturate  UpperLimit=5  LowerLimit=-5
  Scope : Scope
  Sum1 : Sum  Inputs=|++
  Switch : Switch  Criteria=u2 > Threshold  SaturateOnIntegerOverflow=off  InputSameDT=off
  ABS Torque OUT : Outport
  wires:
  Constant1/1 -> Switch/2, Switch/1
  Switch/1 -> Sum1/2  "Ref Slip Ratio"
  Constant2/1 -> Switch/3
  Sum1/1 -> PID Controller/1  "Slip Ratio Delta"
  Torque IN/1 -> Product/1  "Torque IN"
  Product/1 -> ABS Torque OUT/1  "Torq OUT"
  Slip_Ratio/1 -> Gain/1  "Slip Ratio"
  PID Controller/1 -> Scope/1, Saturation/1
  Saturation/1 -> Product/2
  Gain/1 -> Sum1/1

== system Rebuild/Main/Powertrain/Motors/Control Algorithms/ABS1/ABS_RR1 ==
  Torque IN : Inport
  Slip_Ratio : Inport  Port=2
  Constant1 : Constant  Value=0.15
  Constant2 : Constant  Value=0.3
  Gain : Gain  Gain=-1
  PID Controller : slpidlib/PID Controller  Controller=PI  Form=Ideal  TimeDomain=Continuous-time  UseExternalTs=off  SampleTime=-1  IntegratorMethod=Forward Euler  FilterMethod=Forward Euler  ControllerParametersSource=internal  P=50  I=2.5  UseKiTs=on  D=1  UseExternalDerivativeSource=off  N=100  UseFilter=on  TunerSelectOption=Transfer Function Based (PID Tuner App)  InitialConditionSource=internal  InitialConditionForIntegrator=0  InitialConditionForFilter=0  DifferentiatorICPrevScaledInput=0  ExternalReset=none  TrackingMode=off  Kt=1  LimitOutput=off  SatLimitsSource=internal  UpperSaturationLimit=inf  LowerSaturationLimit=-inf  LinearizeAsGain=on  AntiWindupMode=none  Kb=1  LimitIntegrator=off  UpperIntegratorSaturationLimit=inf  LowerIntegratorSaturationLimit=-inf  POutMin=[]  POutMax=[]  IOutMin=[]  IOutMax=[]  DOutMin=[]  DOutMax=[]  NOutMin=[]  NOutMax=[]  SumOutMin=[]  SumOutMax=[]  SaturationOutMin=[]  SaturationOutMax=[]  PParamMin=[]  PParamMax=[]  IParamMin=[]  IParamMax=[]  DParamMin=[]  DParamMax=[]  NParamMin=[]  NParamMax=[]  KbParamMin=[]  KbParamMax=[]  KtParamMin=[]  KtParamMax=[]  KbOutMin=[]  KbOutMax=[]  KtOutMin=[]  KtOutMax=[]  IntegratorOutMin=[]  IntegratorOutMax=[]  FilterOutMin=[]  FilterOutMax=[]  SumI1OutMin=[]  SumI1OutMax=[]  SumI2OutMin=[]  SumI2OutMax=[]  SumI3OutMin=[]  SumI3OutMax=[]  SumI4OutMin=[]  SumI4OutMax=[]  SumDOutMin=[]  SumDOutMax=[]  DifferentiatorOutMin=[]  DifferentiatorOutMax=[]  FilterDiffOutCoefMin=[]  FilterDiffOutCoefMax=[]  ReciprocalOutMin=[]  ReciprocalOutMax=[]  SumDenOutMin=[]  SumDenOutMax=[]  SumNumOutMin=[]  SumNumOutMax=[]  DivideOutMin=[]  DivideOutMax=[]  UdiffTsProdOutMin=[]  UdiffTsProdOutMax=[]  NTsProdOutMin=[]  NTsProdOutMax=[]  UintegralTsProdOutMin=[]  UintegralTsProdOutMax=[]  UngainTsProdOutMin=[]  UngainTsProdOutMax=[]  ClampingZeroOutDataTypeStr=Inherit: Inherit via back propagation  ClampingZeroOutMin=[]  ClampingZeroOutMax=[]  FilterDenConstantOutDataTypeStr=Inherit: Inherit via back propagation  FilterDenConstantOutMin=[]  FilterDenConstantOutMax=[]  PCopyOutDataTypeStr=Inherit: Inherit via back propagation  PCopyOutMin=[]  PCopyOutMax=[]  NCopyOutDataTypeStr=Inherit: Inherit via back propagation  NCopyOutMin=[]  NCopyOutMax=[]  IntegratorContinuousStateAttributes=''  IntegratorStateMustResolveToSignalObject=off  IntegratorRTWStateStorageClass=Auto  FilterContinuousStateAttributes=''  FilterStateMustResolveToSignalObject=off  FilterRTWStateStorageClass=Auto  ParallelPVariant=Passthrough  IdealPVariant=InternalParameters  IVariant=InternalParameters  DVariant=Disabled  IntegratorVariant=Continuous  SatVariant=Disabled  AWVariant=Passthrough  PCopyVariant=Disabled  TRVariant=Disabled  FdbkBlocksVariant=Forward  IdealPFdbkVariant=Disabled  SatFdbkVariant=Disabled  DerivativeFilterVariant=Disabled  NVariant=Disabled  NCopyVariant=Disabled_SignalSpec  FilterICVariant=Disabled  IntegratorICVariant=InternalICs  ExternalResetVariant=Disabled  TRSumVariant=Passthrough  SumFdbkVariant=Disabled  SumVariant=Sum_PI  TsampFilterVariant=InternalTs  TsampNgainVariant=Passthrough  TsampIntegralVariant=Disabled_SignalSpec  ExternalSaturationOutDataTypeStr=Inherit: Same as second input  DerivativeSourceVariant=Disabled  PreIntVariant=InternalPreInt
  Product : Product
  Saturation : Saturate  UpperLimit=5  LowerLimit=-5
  Scope : Scope
  Sum1 : Sum  Inputs=|++
  Switch : Switch  Criteria=u2 > Threshold  SaturateOnIntegerOverflow=off  InputSameDT=off
  ABS Torque OUT : Outport
  wires:
  Constant1/1 -> Switch/2, Switch/1
  Switch/1 -> Sum1/2  "Ref Slip Ratio"
  Constant2/1 -> Switch/3
  Sum1/1 -> PID Controller/1  "Slip Ratio Delta"
  Torque IN/1 -> Product/1  "Torque IN"
  Product/1 -> ABS Torque OUT/1  "Torq OUT"
  Slip_Ratio/1 -> Gain/1  "Slip Ratio"
  PID Controller/1 -> Scope/1, Saturation/1
  Saturation/1 -> Product/2
  Gain/1 -> Sum1/1

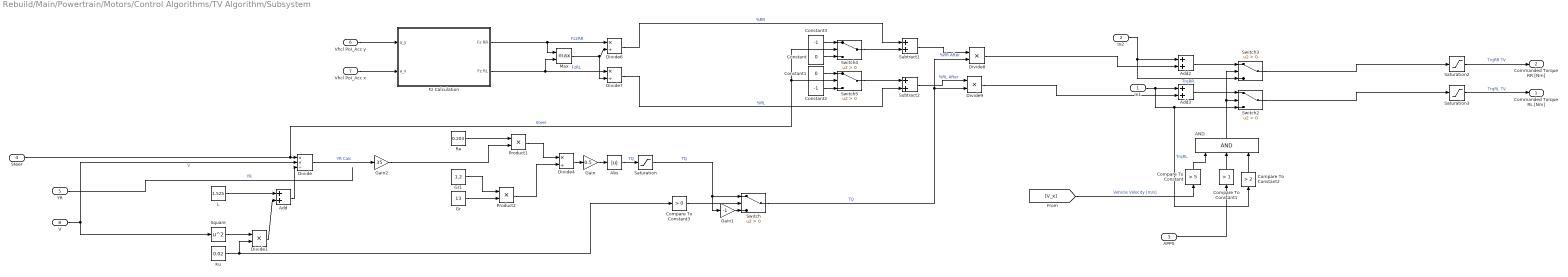
== system Rebuild/Main/Powertrain/Motors/Control Algorithms/TV Algorithm/Subsystem ==
  In1 : Inport
  In2 : Inport  Port=2
  APPS : Inport  Port=3
  Steer : Inport  Port=4
  YR : Inport  Port=5
  Vhcl PoI_Acc y : Inport  Port=6
  Vhcl PoI_Acc x : Inport  Port=7
  V : Inport  Port=8
  AND : Logic  Inputs=3  IconShape=distinctive  AllPortsSameDT=off  OutDataTypeStr=boolean
  Abs : Abs  SaturateOnIntegerOverflow=off
  Add : Sum
  Add2 : Sum
  Add3 : Sum
  Compare To Constant : simulink/Logic and Bit Operations/Compare To Constant  relop=>  const=5  OutDataTypeStr=boolean
  Compare To Constant1 : simulink/Logic and Bit Operations/Compare To Constant  relop=>  const=1  OutDataTypeStr=boolean
  Compare To Constant2 : simulink/Logic and Bit Operations/Compare To Constant  relop=>  const=2  OutDataTypeStr=boolean
  Compare To Constant3 : simulink/Logic and Bit Operations/Compare To Constant  relop=>  const=0  OutDataTypeStr=boolean
  Constant : Constant  Value=0
  Constant1 : Constant  Value=0
  Constant2 : Constant  Value=-1
  Constant3 : Constant  Value=-1
  Divide : Product  Inputs=**/
  Divide1 : Product  Inputs=**
  Divide4 : Product  Inputs=*/
  Divide6 : Product  Inputs=*/
  Divide7 : Product  Inputs=*/
  Divide8 : Product  Inputs=**
  Divide9 : Product  Inputs=**
  Fz Calculation : Subsystem
  Gain : Gain  Gain=0.5
  Gain1 : Gain  Gain=-1
  Gain2 : Gain  Gain=35
  Gr : Constant  Value=13
  Gr1 : Constant  Value=1.2
  Ku : Constant  Value=0.02
  L : Constant  Value=1.525
  Max : MinMax  Function=max  Inputs=2
  Product1 : Product
  Product2 : Product
  Re : Constant  Value=0.203
  Saturation : Saturate  UpperLimit=8  LowerLimit=0
  Saturation2 : Saturate  UpperLimit=Max_Torque  LowerLimit=0
  Saturation3 : Saturate  UpperLimit=Max_Torque  LowerLimit=0
  Square : Math  Operator=square
  Subtract1 : Sum
  Subtract2 : Sum
  Switch{,2..5} (5 alike) : Switch  Criteria=u2 > Threshold  SaturateOnIntegerOverflow=off  InputSameDT=off
  Commanded Torque RL [Nm] : Outport
  Commanded Torque RR [Nm] : Outport  Port=2
  wires:
  Max/1 -> Divide7/2, Divide6/2
  Divide9/1 -> Add3/2
  L/1 -> Add/1
  Steer/1 -> Switch4/2, Switch5/2, Divide/1  "Steer"
  In1/1 -> Compare To Constant2/1, Switch2/3, Add3/1  "TrqRL"
  Vhcl PoI_Acc y/1 -> Fz Calculation/1(a_y)
  Divide8/1 -> Add2/2
  Divide6/1 -> Subtract1/1  "%RR"
  In2/1 -> Switch3/3, Add2/1  "TrqRR"
  Vhcl PoI_Acc x/1 -> Fz Calculation/2(a_x)
  Divide4/1 -> Gain/1
  Add3/1 -> Switch2/1
  Divide7/1 -> Subtract2/2  "%RL"
  Divide1/1 -> Add/2
  Ku/1 -> Compare To Constant3/1, Divide1/2
  Add/1 -> Divide/3
  Divide/1 -> Gain2/1  "YR Calc"
  Fz Calculation/2(Fz RL) -> Max/2, Divide7/1  "FzRL"
  Square/1 -> Divide1/1
  Saturation2/1 -> Commanded Torque RR [Nm]/1  "TrqRR TV"
  Saturation3/1 -> Commanded Torque RL [Nm]/1  "TrqRL TV"
  Re/1 -> Product1/1
  Product1/1 -> Divide4/1
  Gr/1 -> Product2/2
  Gain2/1 -> Product1/2
  Switch/1 -> Divide8/2, Divide9/2  "TQ"
  YR/1 -> ?  "YR"
  Gr1/1 -> Product2/1
  Product2/1 -> Divide4/2
  V/1 -> Square/1, Divide/2  "V"
  Gain/1 -> Abs/1
  Add2/1 -> Switch3/1
  [V_x] -> Compare To Constant/1  "Vehicle Velocity [m/s]"
  Compare To Constant/1 -> AND/1
  Compare To Constant1/1 -> AND/2
  APPS/1 -> Compare To Constant1/1
  AND/1 -> Switch2/2, Switch3/2
  Abs/1 -> Saturation/1  "TQ"
  Subtract1/1 -> Divide8/1  "%RR After"
  Subtract2/1 -> Divide9/1  "%RL After"
  Constant2/1 -> Switch5/3
  Switch4/1 -> Subtract1/2
  Switch5/1 -> Subtract2/1
  Constant/1 -> Switch4/3
  Constant1/1 -> Switch5/1
  Constant3/1 -> Switch4/1
  Compare To Constant2/1 -> AND/3
  Switch3/1 -> Saturation2/1
  Switch2/1 -> Saturation3/1
  Compare To Constant3/1 -> Switch/2
  Saturation/1 -> Switch/1, Gain1/1  "TQ"
  Gain1/1 -> Switch/3
  Fz Calculation/1(Fz RR) -> Max/1, Divide6/1  "Fz2RR"

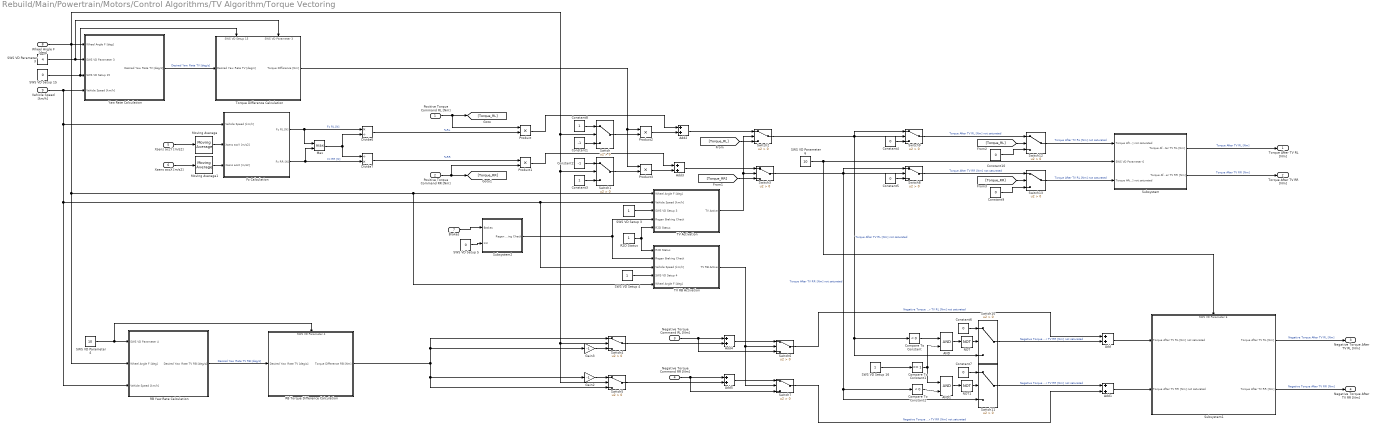
== system Rebuild/Main/Powertrain/Motors/Control Algorithms/TV Algorithm/Torque Vectoring ==
  Positive Torque Command RL [Nm] : Inport
  Positive Torque Command RR [Nm] : Inport  Port=2
  Negative Torque Command RL [Nm] : Inport  Port=3
  Negative Torque Command RR [Nm] : Inport  Port=4
  Xsens accY [m/s2] : Inport  Port=5
  Xsens accX [m/s2] : Inport  Port=6
  Brakes : Inport  Port=7
  Wheel Angle F [deg] : Inport  Port=8
  Vehicle Speed [km/h] : Inport  Port=9
  AND : Logic  IconShape=distinctive  AllPortsSameDT=off  OutDataTypeStr=boolean
  AND1 : Logic  IconShape=distinctive  AllPortsSameDT=off  OutDataTypeStr=boolean
  Add{,1..5} (6 alike) : Sum
  Compare To Constant : simulink/Logic and Bit Operations/Compare To Constant  relop=<  const=0  OutDataTypeStr=boolean
  Compare To Constant1 : simulink/Logic and Bit Operations/Compare To Constant  relop===  const=1  OutDataTypeStr=boolean
  Compare To Constant2 : simulink/Logic and Bit Operations/Compare To Constant  relop=<  const=0  OutDataTypeStr=boolean
  Constant1 : Constant  Value=-1
  Constant{4..7,9..10} (6 alike) : Constant  Value=0
  Constant2 : Constant  Value=-1
  Constant3 : Constant
  Constant8 : Constant
  Divide6 : Product  Inputs=*/
  Divide7 : Product  Inputs=/*
  Fz Calculation : Subsystem
  Gain2 : Gain  Gain=-1
  Gain3 : Gain  Gain=-1
  Max : MinMax  Function=max  Inputs=2
  Moving Average : dspstat3/Moving Average  Method=Sliding window  ForgettingFactorPort=off  SpecifyWindowLength=on  WindowLength=4  OverlapLength=3  AllowArbitraryInputLength=off  ForgettingFactor=0.9  SimulateUsing=Code generation
  Moving Average1 : dspstat3/Moving Average  Method=Sliding window  ForgettingFactorPort=off  SpecifyWindowLength=on  WindowLength=4  OverlapLength=3  AllowArbitraryInputLength=off  ForgettingFactor=0.9  SimulateUsing=Code generation
  NOT : Logic  Operator=NOT  IconShape=distinctive  AllPortsSameDT=off  OutDataTypeStr=boolean
  NOT1 : Logic  Operator=NOT  IconShape=distinctive  AllPortsSameDT=off  OutDataTypeStr=boolean
  Product{,1..3} (4 alike) : Product
  R2D Status : Constant
  RB Torque Difference Calculation : Subsystem
      settings: PortSchema="{\"entries\":[{\"content\":{\"sides\":[{\"content\":{\"connectorIds\":[\"In1\"]},\"type\":\"ConnectorPlacement.EquallySpacedRectSide\",\"uuid\":\"fa4973ad-a32f-4095-ab0b-cea383016739\"},{\"content\":{\"connectorIds\":[\"Out1\"],\"side\":\"RIGHT\"},\"type\":\"ConnectorPlacement.EquallySpacedRectSide\",\"uuid\":\"939e1308-df81-4bd9-8a82-65ce288053d3\"},{\"content\":{\"connectorIds\":[\"In2\"],\"side\":\"TOP\"},\"type\":\"ConnectorPlacement.EquallySpacedRectSide\",\"uuid\":\"fc465ebf-5b67-4318-901e-ca5dd36e3a85\"}]},\"type\":\"ConnectorPlacement.EquallySpacedConnector\",\"uuid\":\"4f087700-9ed6-4341-833d-4cc93a86ad38\"}],\"packageUris\":[\"http://schema.mathworks.com/mf0/Connector/R2020b\"],\"version\":\"1.0\"}"
  RB Yaw Rate Calculation : Subsystem
  SWS VD Parameter 3 : Constant  Value=4
  SWS VD Parameter 4 : Constant  Value=10
  SWS VD Parameter 6 : Constant  Value=10
  SWS VD Setup 15 : Constant  Value=0
  SWS VD Setup 16 : Constant
  SWS VD Setup 3 : Constant
  SWS VD Setup 4 : Constant
  SWS VD Setup 5 : Constant  Value=0
  Subsystem : Subsystem
  Subsystem1 : Subsystem
      settings: PortSchema="{\"entries\":[{\"content\":{\"sides\":[{\"content\":{\"connectorIds\":[\"In1\",\"In2\"]},\"type\":\"ConnectorPlacement.EquallySpacedRectSide\",\"uuid\":\"3056adb4-125a-41ff-b8f3-94632bed0e59\"},{\"content\":{\"connectorIds\":[\"Out1\",\"Out2\"],\"side\":\"RIGHT\"},\"type\":\"ConnectorPlacement.EquallySpacedRectSide\",\"uuid\":\"828b5026-b9f0-47a0-9847-e54771aaad3f\"},{\"content\":{\"connectorIds\":[\"In3\"],\"side\":\"TOP\"},\"type\":\"ConnectorPlacement.EquallySpacedRectSide\",\"uuid\":\"5565ffc5-94d3-407e-898e-a464d97134f1\"}]},\"type\":\"ConnectorPlacement.EquallySpacedConnector\",\"uuid\":\"ef74bfd7-20f4-4a9c-8af2-e6f991f2b9d8\"}],\"packageUris\":[\"http://schema.mathworks.com/mf0/Connector/R2020b\"],\"version\":\"1.0\"}"
  Subsystem2 : Subsystem
  Switch{,1..13} (14 alike) : Switch  Criteria=u2 > Threshold  SaturateOnIntegerOverflow=off  InputSameDT=off
  TV Activation : Subsystem
  TV RB Activation : Subsystem
  Torque Difference Calculation : Subsystem
      settings: PortSchema="{\"entries\":[{\"content\":{\"sides\":[{\"content\":{\"connectorIds\":[\"In1\"]},\"type\":\"ConnectorPlacement.EquallySpacedRectSide\",\"uuid\":\"fa4973ad-a32f-4095-ab0b-cea383016739\"},{\"content\":{\"connectorIds\":[\"Out1\"],\"side\":\"RIGHT\"},\"type\":\"ConnectorPlacement.EquallySpacedRectSide\",\"uuid\":\"939e1308-df81-4bd9-8a82-65ce288053d3\"},{\"content\":{\"connectorIds\":[\"In2\",\"In3\"],\"side\":\"TOP\"},\"type\":\"ConnectorPlacement.EquallySpacedRectSide\",\"uuid\":\"fc465ebf-5b67-4318-901e-ca5dd36e3a85\"}]},\"type\":\"ConnectorPlacement.EquallySpacedConnector\",\"uuid\":\"4f087700-9ed6-4341-833d-4cc93a86ad38\"}],\"packageUris\":[\"http://schema.mathworks.com/mf0/Connector/R2020b\"],\"version\":\"1.0\"}"
  Yaw Rate Calculation : Subsystem
  Torque After TV RL [Nm] : Outport
  Torque After TV RR [Nm] : Outport  Port=2
  Negative Torque After TV RL [Nm] : Outport  Port=3
  Negative Torque After TV RR [Nm] : Outport  Port=4
  wires:
  Moving Average1/1 -> Fz Calculation/3(Xsens accX [m/s2])
  R2D Status/1 -> TV RB Activation/1(R2D Status), TV Activation/5(R2D Status)
  TV Activation/1(TV Active) -> Switch2/2, Switch3/2
  Subsystem/2(Torque After TV RR [Nm]) -> Torque After TV RR [Nm]/1  "Torque After TV RR [Nm]"
  Yaw Rate Calculation/1(Desired Yaw Rate TV [deg/s]) -> Torque Difference Calculation/1(Desired Yaw Rate TV [deg/s])  "Desired Yaw Rate TV [deg/s]"
  Fz Calculation/1(Fz RL [N]) -> Divide6/1, Max/1  "Fz RL [N]"
  Xsens accY [m/s2]/1 -> Moving Average/1
  Subsystem/1(Torque After TV RL [Nm]) -> Torque After TV RL [Nm]/1  "Torque After TV RL [Nm]"
  SWS VD Setup 3/1 -> TV Activation/3(SWS VD Setup 3)
  Divide6/1 -> Product/2  "%RL"
  Switch3/1 -> Switch8/2, Compare To Constant2/1, Switch11/3, Switch8/1  "Torque After TV RR [Nm] not saturated"
  Wheel Angle F [deg]/1 -> RB Yaw Rate Calculation/2(Wheel Angle F [deg]), TV RB Activation/5(Wheel Angle F [deg]), TV Activation/1(Wheel Angle F [deg]), Switch5/2, Switch4/2, Switch1/2, Switch/2, Yaw Rate Calculation/1(Wheel Angle F [deg])
  Xsens accX [m/s2]/1 -> Moving Average1/1
  SWS VD Parameter 3/1 -> Yaw Rate Calculation/2(SWS VD Parameter 3), Torque Difference Calculation/3(SWS VD Parameter 3)
  Divide7/1 -> Product1/1  "%RR"
  Switch2/1 -> Compare To Constant/1, Switch10/3, Switch9/1, Switch9/2  "Torque After TV RL [Nm] not saturated"
  Max/1 -> Divide6/2, Divide7/1
  Vehicle Speed [km/h]/1 -> Fz Calculation/1(Vehicle Speed [km/h]), TV RB Activation/3(Vehicle Speed [km/h]), TV Activation/2(Vehicle Speed [km/h]), RB Yaw Rate Calculation/3(Vehicle Speed [km/h]), Yaw Rate Calculation/4(Vehicle Speed [km/h])
  Fz Calculation/2(Fz RR [N]) -> Max/2, Divide7/2  "Fz RR [N]"
  Moving Average/1 -> Fz Calculation/2(Xsens accY [m/s2])
  SWS VD Parameter 6/1 -> Subsystem1/3(SWS VD Parameter 6), Subsystem/2(SWS VD Parameter 6)
  Torque Difference Calculation/1(Torque Difference [Nm]) -> Product3/1, Product2/1
  Negative Torque Command RL [Nm]/1 -> Switch6/3, Add4/1
  Switch4/1 -> Add4/2
  Switch5/1 -> Add5/2
  Negative Torque Command RR [Nm]/1 -> Add5/1, Switch7/3
  Add4/1 -> Switch6/1
  TV RB Activation/1(TV RB Active) -> Switch6/2, Switch7/2
  Add5/1 -> Switch7/1
  SWS VD Setup 4/1 -> TV RB Activation/4(SWS VD Setup 4)
  Subsystem1/1(Torque After TV RL [Nm]) -> Negative Torque After TV RL [Nm]/1  "Negative Torque After TV RL [Nm]"
  Subsystem1/2(Torque After TV RR [Nm]) -> Negative Torque After TV RR [Nm]/1  "Negative Torque After TV RR [Nm]"
  Gain2/1 -> Switch5/1
  Gain3/1 -> Switch4/3
  Positive Torque Command RL [Nm]/1 -> [Torque_RL], Product/1
  Positive Torque Command RR [Nm]/1 -> [Torque_RR], Product1/2
  Constant8/1 -> Switch/1
  Constant1/1 -> Switch/3
  Constant2/1 -> Switch1/1
  Constant3/1 -> Switch1/3
  Switch/1 -> Product2/2
  Switch1/1 -> Product3/2
  [Torque_RR] -> Switch3/3
  [Torque_RL] -> Switch2/3
  Constant4/1 -> Switch9/3
  Constant5/1 -> Switch8/3
  Switch9/1 -> Switch12/1  "Torque After TV RL [Nm] not saturated"
  Switch8/1 -> Switch13/1  "Torque After TV RR [Nm] not saturated"
  Constant6/1 -> Switch10/1
  Add/1 -> Subsystem1/1(Torque After TV RL [Nm] not saturated)
  Constant7/1 -> Switch11/1
  Add1/1 -> Subsystem1/2(Torque After TV RR [Nm] not saturated)
  Add2/1 -> Switch2/1
  Product2/1 -> Add2/2
  Product/1 -> Add2/1
  Product1/1 -> Add3/1
  Product3/1 -> Add3/2
  Add3/1 -> Switch3/1
  SWS VD Setup 15/1 -> Torque Difference Calculation/2(SWS VD Setup 15), Yaw Rate Calculation/3(SWS VD Setup 15)
  [Torque_RL] -> Switch12/2
  [Torque_RR] -> Switch13/2
  Constant9/1 -> Switch13/3
  Constant10/1 -> Switch12/3
  Switch12/1 -> Subsystem/1(Torque After TV RL [Nm] not saturated)  "Torque After TV RL [Nm] not saturated"
  Switch13/1 -> Subsystem/3(Torque After TV RR [Nm] not saturated)  "Torque After TV RL [Nm] not saturated"
  RB Yaw Rate Calculation/1(Desired Yaw Rate TV RB [deg/s]) -> RB Torque Difference Calculation/1(Desired Yaw Rate TV [deg/s])  "Desired Yaw Rate TV RB [deg/s]"
  RB Torque Difference Calculation/1(Torque Difference RB [Nm]) -> Switch4/1, Gain3/1, Switch5/3, Gain2/1
  Subsystem2/1(Regen Braking Check) -> TV Activation/4(Regen Braking Check), TV RB Activation/2(Regen Braking Check)
  SWS VD Parameter 4/1 -> RB Torque Difference Calculation/2(SWS VD Parameter 4), RB Yaw Rate Calculation/1(SWS VD Parameter 4)
  Compare To Constant/1 -> AND/1
  Compare To Constant1/1 -> AND/2, AND1/1
  SWS VD Setup 16/1 -> Compare To Constant1/1
  Switch11/1 -> Add1/1  "Negative Torque After TV RR [Nm] not saturated"
  Switch10/1 -> Add/2  "Negative Torque After TV RR [Nm] not saturated"
  AND/1 -> NOT/1
  AND1/1 -> NOT1/1
  Compare To Constant2/1 -> AND1/2
  Switch6/1 -> Add/1  "Negative Torque After TV RL [Nm] not saturated"
  Switch7/1 -> Add1/2  "Negative Torque After TV RR [Nm] not saturated"
  NOT/1 -> Switch10/2
  NOT1/1 -> Switch11/2
  SWS VD Setup 5/1 -> Subsystem2/2(In3)
  Brakes/1 -> Subsystem2/1(Brakes)

== system Rebuild/Main/Powertrain/Motors/Control Algorithms/TV Algorithm/Subsystem/Fz Calculation ==
  a_y : Inport
  a_x : Inport  Port=2
  Add : Sum
  Add1 : Sum
  Fz RL Calculation : Subsystem
  Fz RR Calculation : Subsystem
  Gain : Gain  Gain=0.5
  Gain1 : Gain  Gain=air_density
  Gain2 : Gain  Gain=1/2
  Gain3 : Gain  Gain=Cl
  Gain4 : Gain  Gain=A
  Gain5 : Gain  Gain=aero_balance
  Square : Math  Operator=square
  Fz RR : Outport
  Fz RL : Outport  Port=2
  wires:
  a_x/1 -> Fz RL Calculation/2(a_x), Fz RR Calculation/2(a_x)  "ax"
  a_y/1 -> Fz RL Calculation/1(a_y), Fz RR Calculation/1(a_y)  "ay"
  Gain2/1 -> Gain3/1
  Square/1 -> Gain4/1
  Gain3/1 -> Gain5/1  "Downforce [N]"
  Gain1/1 -> Gain2/1
  Gain4/1 -> Gain1/1
  [V_x] -> Square/1  "Vehicle Velocity [m/s]"
  Add/1 -> Fz RR/1  "Fz RR"
  Fz RR Calculation/1(Fz RR) -> Add/2
  Gain5/1 -> Gain/1  "Downforce Rear"
  Gain/1 -> Add1/1, Add/1
  Fz RL Calculation/1(Fz RL) -> Add1/2
  Add1/1 -> Fz RL/1  "Fz RL"
